simulink model "einMassenSchwinger"  (R2017b)
settings: Solver=VariableStepAuto  StartTime=0.0  StopTime=t_max  RelTol=1e-3
values from neighbouring files (symbols this model uses):
  c = 10    [Aufgabe2_parameterInit.m]
  d = .5    (= 0.5)    [Aufgabe2_parameterInit.m]
  m = 1    [Aufgabe2_parameterInit.m]
  y0 = 0    [Aufgabe2_parameterInit.m]
  yDot0 = 0    [Aufgabe2_parameterInit.m]
settings Model: Creator=ucelm  LastModifiedBy=jens
settings CodeAppCC: StateflowObjectComments=on

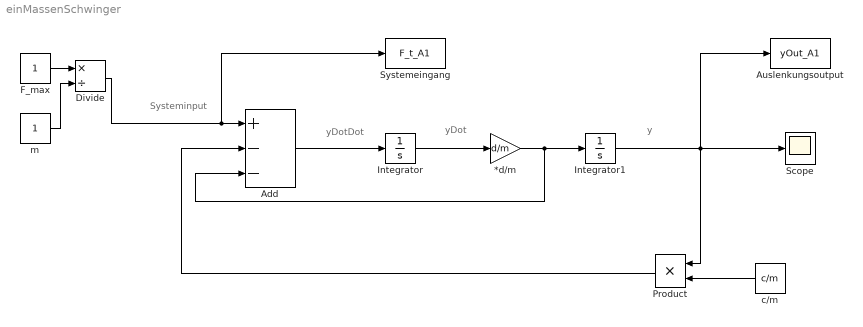
== system einMassenSchwinger ==
  note: yDotDot
  note: y
  note: yDot
  note: Systeminput
  *d/m : Gain  Gain=d/m
  Add : Sum  Inputs=+--
  Auslenkungsoutput : ToWorkspace  VariableName=yOut_A1  SaveFormat=Timeseries  SampleTime=-1
  Divide : Product  Inputs=*/
  F_max : Constant
  Integrator : Integrator  InitialCondition=yDot0
  Integrator1 : Integrator  InitialCondition=y0
  Product : Product
  Scope : Scope
  Systemeingang : ToWorkspace  VariableName=F_t_A1  SaveFormat=Timeseries  SampleTime=-1
  c/m : Constant  Value=c/m
  m : Constant
  wires:
  *d/m/1 -> Add/3, Integrator1/1
  Integrator1/1 -> Auslenkungsoutput/1, Product/1, Scope/1
  c/m/1 -> Product/2
  Add/1 -> Integrator/1
  F_max/1 -> Divide/1
  m/1 -> Divide/2
  Integrator/1 -> *d/m/1
  Divide/1 -> Systemeingang/1, Add/1
  Product/1 -> Add/2
